simulink model "p5"  (R2021b)
settings: Solver=VariableStepAuto  StartTime=0.0  StopTime=10.0  RelTol=1e-3
values from neighbouring files (symbols this model uses):
  A = [0 -0.378002311941 0 18.900115597 1 0 0 0 0 7.01473716863 0 -0.379715574203 ... (16 elements, 4x4)]    [Parameters.mat]
  A_estimator = [-12.5867377374 -54.4559016515 -11.7802838218 0.356524579344 1 0 0 0 0 7.01473716863 0 -0.379715574203 ... (16 elements, 4x4)]    [Parameters.mat]
  B = [0 -0.0699290719413 0 3.49645359707]    [Parameters.mat]
  cx = [1 0 0 0]    [Parameters.mat]
  k_fast = [18149.2945377 2839.00304412 1519.94169463 86.0344853723]    [Parameters.mat]
  k_slow = [20.7523551145 9.40402411533 21.9918477145 2.35791844149]    [Parameters.mat]
  L = [12.5867377374 54.0778993395 11.7802838218 18.5435910177]    [Parameters.mat]
  p_f = 18143.8890275    [Parameters.mat]
  p_s = 15.3468449104    [Parameters.mat]
settings Model: Creator=mahya  LastModifiedBy=mahya

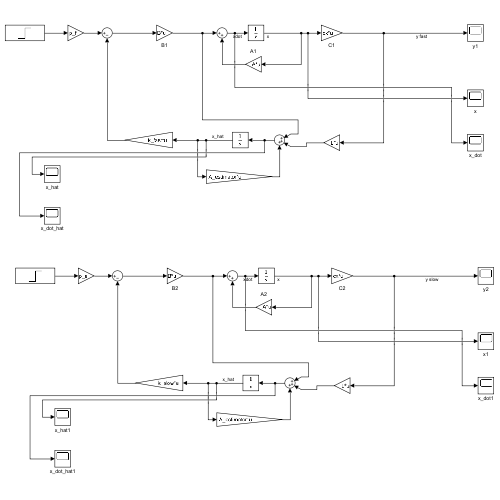
[thumbnail: Simulink's stored preview of the top-level diagram]
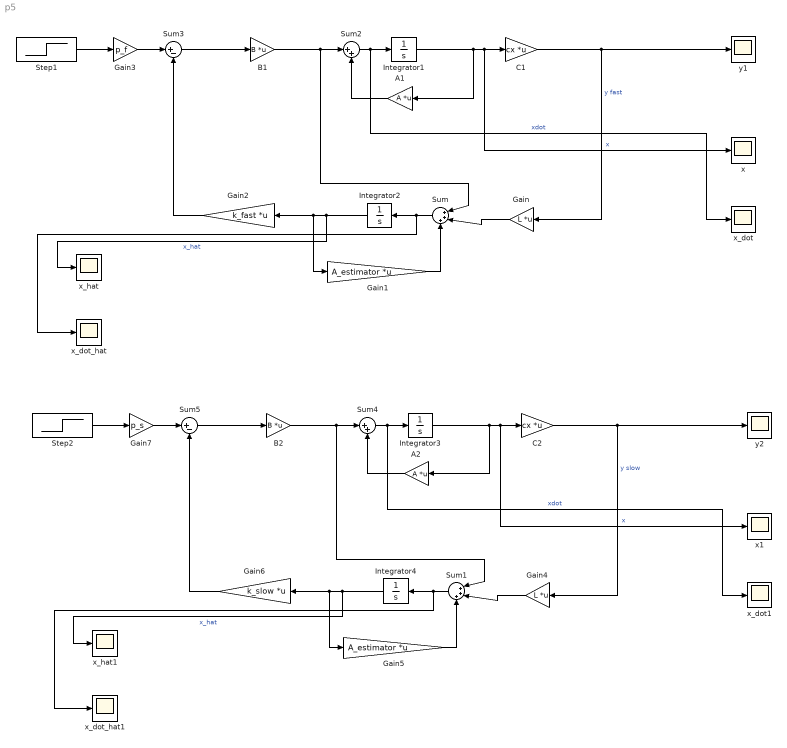
== system p5 ==
  A1 : Gain  Gain=A  Multiplication=Matrix(K*u)
  A2 : Gain  Gain=A  Multiplication=Matrix(K*u)
  B1 : Gain  Gain=B  Multiplication=Matrix(K*u)
  B2 : Gain  Gain=B  Multiplication=Matrix(K*u)
  C1 : Gain  Gain=cx  Multiplication=Matrix(K*u)
  C2 : Gain  Gain=cx  Multiplication=Matrix(K*u)
  Gain : Gain  Gain=L  Multiplication=Matrix(K*u)
  Gain1 : Gain  Gain=A_estimator  Multiplication=Matrix(K*u)
  Gain2 : Gain  Gain=k_fast  Multiplication=Matrix(K*u)
  Gain3 : Gain  Gain=p_f
  Gain4 : Gain  Gain=L  Multiplication=Matrix(K*u)
  Gain5 : Gain  Gain=A_estimator  Multiplication=Matrix(K*u)
  Gain6 : Gain  Gain=k_slow  Multiplication=Matrix(K*u)
  Gain7 : Gain  Gain=p_s
  Integrator{1..4} (4 alike) : Integrator  InitialCondition=[0 0 0 0]
  Step1 : Step  Time=0  SampleTime=0
  Step2 : Step  Time=0  SampleTime=0
  Sum : Sum  Inputs=|+++
  Sum1 : Sum  Inputs=|+++
  Sum2 : Sum  Inputs=|++
  Sum3 : Sum  Inputs=|+-
  Sum4 : Sum  Inputs=|++
  Sum5 : Sum  Inputs=|+-
  x : Scope
  x1 : Scope
  x_dot : Scope
  x_dot1 : Scope
  x_dot_hat : Scope
  x_dot_hat1 : Scope
  x_hat : Scope
  x_hat1 : Scope
  y1 : Scope
  y2 : Scope
  wires:
  Gain3/1 -> Sum3/1
  Integrator1/1 -> A1/1, x/1, C1/1  "x"
  C1/1 -> Gain/1, y1/1  "y fast"
  B1/1 -> Sum2/1, Sum/1
  Step1/1 -> Gain3/1
  Sum2/1 -> x_dot/1, Integrator1/1  "xdot"
  Sum3/1 -> B1/1
  A1/1 -> Sum2/2
  Gain/1 -> Sum/2
  Sum/1 -> x_dot_hat/1, Integrator2/1
  Integrator2/1 -> x_hat/1, Gain1/1, Gain2/1  "x_hat"
  Gain2/1 -> Sum3/2
  Gain1/1 -> Sum/3
  Gain5/1 -> Sum1/3
  Gain6/1 -> Sum5/2
  Sum5/1 -> B2/1
  Sum4/1 -> x_dot1/1, Integrator3/1  "xdot"
  C2/1 -> Gain4/1, y2/1  "y slow"
  A2/1 -> Sum4/2
  Integrator4/1 -> x_hat1/1, Gain5/1, Gain6/1  "x_hat"
  Integrator3/1 -> A2/1, x1/1, C2/1  "x"
  Step2/1 -> Gain7/1
  Gain4/1 -> Sum1/2
  B2/1 -> Sum4/1, Sum1/1
  Gain7/1 -> Sum5/1
  Sum1/1 -> x_dot_hat1/1, Integrator4/1
